simulink model "P2_Ec_Diferencial_A_Modelo_Bloques"  (R2021a)
settings: Solver=ode4  StartTime=0.0  StopTime=10  FixedStep=0.001  RelTol=1e-3
values from neighbouring files (symbols this model uses):
  b = 3    [P2_ED_A_Modelo_Bloques.m]
  k = 1    [P2_ED_A_Modelo_Bloques.m]
  m = 1    [P2_ED_A_Modelo_Bloques.m]
settings Model: Creator=diego  LastModifiedBy=diego
settings SolverCC: AlgebraicLoopSolver=TrustRegion
settings DataIOCC: ReturnWorkspaceOutputs=off
settings DebuggingCC: SFMachineParentedDataDiag=warning  ArithmeticOperatorsInVariantConditions=warning
settings SFSimCC: CustomCodeUndefinedFunction=UseInterfaceOnly

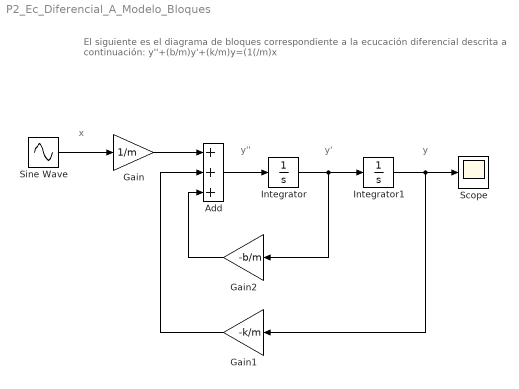
== system P2_Ec_Diferencial_A_Modelo_Bloques ==
  note: y'
  note: y''
  note: y
  note: x
  note: El siguiente es el diagrama de bloques correspondiente a la ecucación diferencial descrita a continuación:
      | y''+(b/m)y'+(k/m)y=(1(/m)x
  Add : Sum  Inputs=+++
  Gain : Gain  Gain=1/m
  Gain1 : Gain  Gain=-k/m
  Gain2 : Gain  Gain=-b/m
  Integrator : Integrator
  Integrator1 : Integrator  InitialCondition=1
  Scope : Scope
  Sine Wave : Sin  Amplitude=2  Frequency=8*pi  Phase=pi/2  SampleTime=0
  wires:
  Gain2/1 -> Add/3
  Gain1/1 -> Add/2
  Gain/1 -> Add/1
  Add/1 -> Integrator/1
  Integrator/1 -> Gain2/1, Integrator1/1
  Integrator1/1 -> Gain1/1, Scope/1
  Sine Wave/1 -> Gain/1
